simulink model "MultiAgentNewtonian"  (R2017a)
settings: Solver=ode1  StartTime=0.0  StopTime=50  FixedStep=tstep  RelTol=1e-3
InitFcn:
  | initSim;
StopFcn:
  | plotSimSolution;
values from neighbouring files (symbols this model uses):
  tstep = 0.1    [initSim.m]
undefined symbols (not defined in the file or in its folder): m, problem
settings Model: Creator=yn15  LastModifiedBy=DAW15
settings OptimizationCC: LifeSpan=inf
settings DebuggingCC: SFUnexpectedBacktrackingDiag=warning  SFNoUnconditionalDefaultTransitionDiag=warning  SFExecutionAtInitializationDiag=none
settings GRTTargetCC: TargetLangStandard=C89/C90 (ANSI)
settings ConfigComp: CovMetricSettings=dw  CovHtmlReporting=on  CovSaveCumulativeToWorkspaceVar=on  CovSaveSingleToWorkspaceVar=on  CovExternalEMLEnable=off

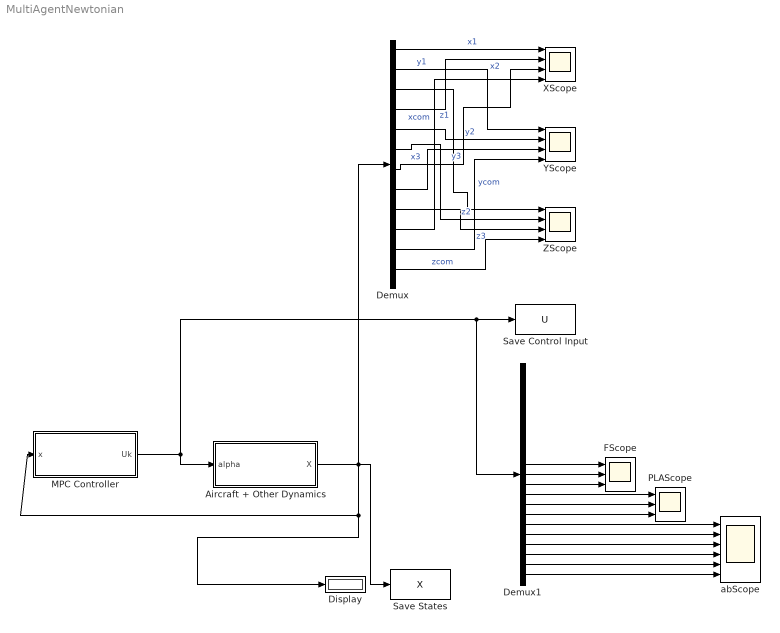
== system MultiAgentNewtonian ==
  Aircraft + Other Dynamics : Subsystem
  Demux : Demux  Outputs=24
  Demux1 : Demux  Outputs=21
  Display : Display
  FScope : Scope  NumInputPorts=3
  "MPC Controller " : Subsystem
  PLAScope : Scope  NumInputPorts=3
  Save Control Input : ToWorkspace  VariableName=U  SampleTime=-1
      settings: Save2DSignal=2-D array (concatenate along first dimension)
  Save States : ToWorkspace  VariableName=X  SaveFormat=Timeseries  SampleTime=-1
  XScope : Scope  NumInputPorts=4
  YScope : Scope  NumInputPorts=4
  ZScope : Scope  NumInputPorts=4
  abScope : Scope  NumInputPorts=6
  wires:
  Aircraft + Other Dynamics/1(X) -> Demux/1, Save States/1, "MPC Controller "/1(x), Display/1
  "MPC Controller "/1(Uk) -> Demux1/1, Save Control Input/1, Aircraft + Other Dynamics/1(alpha)
  Demux/1 -> XScope/1  "x1"
  Demux/3 -> YScope/1  "y1"
  Demux/5 -> ZScope/1  "z1"
  Demux/7 -> XScope/2  "x2"
  Demux/9 -> YScope/2  "y2"
  Demux/11 -> ZScope/2  "z2"
  Demux/13 -> XScope/3  "x3"
  Demux/15 -> YScope/3  "y3"
  Demux/17 -> ZScope/3  "z3"
  Demux/19 -> XScope/4  "xcom"
  Demux/21 -> YScope/4  "ycom"
  Demux/23 -> ZScope/4  "zcom"
  Demux1/10 -> FScope/1
  Demux1/11 -> FScope/2
  Demux1/12 -> FScope/3
  Demux1/13 -> PLAScope/1
  Demux1/14 -> PLAScope/2
  Demux1/15 -> PLAScope/3
  Demux1/16 -> abScope/1
  Demux1/17 -> abScope/2
  Demux1/18 -> abScope/3
  Demux1/19 -> abScope/4
  Demux1/20 -> abScope/5
  Demux1/21 -> abScope/6

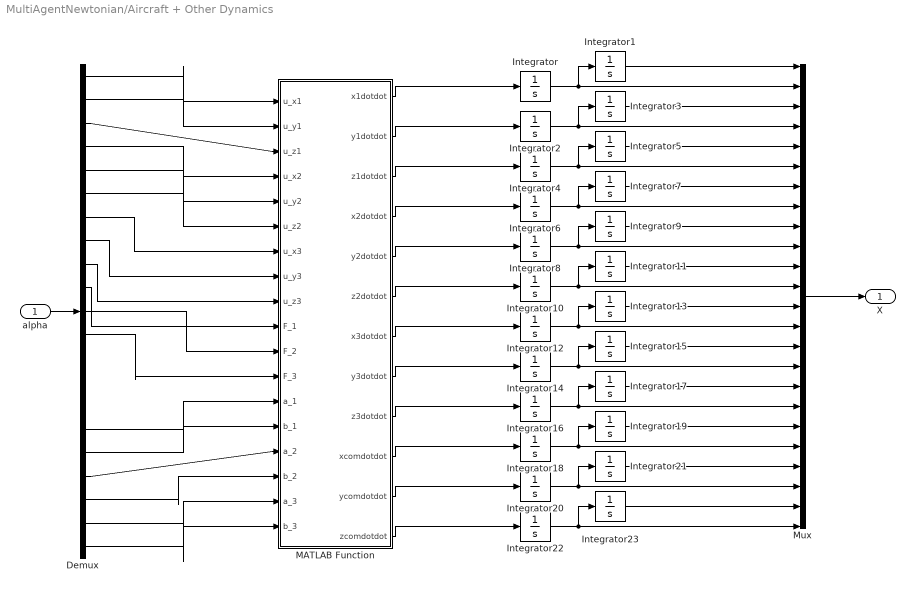
== system MultiAgentNewtonian/Aircraft + Other Dynamics ==
  alpha : Inport
  Demux : Demux  Outputs=21
  Integrator{,1..23} (24 alike) : Integrator
  MATLAB Function : MATLAB Function  TreatAsAtomicUnit=on
  Mux : Mux  Inputs=24
  X : Outport
  wires:
  MATLAB Function/3(z1dotdot) -> Integrator4/1
  MATLAB Function/6(z2dotdot) -> Integrator10/1
  MATLAB Function/9(z3dotdot) -> Integrator16/1
  Integrator/1 -> Mux/2, Integrator1/1
  MATLAB Function/1(x1dotdot) -> Integrator/1
  Integrator2/1 -> Mux/4, Integrator3/1
  Integrator4/1 -> Mux/6, Integrator5/1
  Integrator6/1 -> Mux/8, Integrator7/1
  Integrator8/1 -> Mux/10, Integrator9/1
  Integrator10/1 -> Mux/12, Integrator11/1
  Integrator12/1 -> Mux/14, Integrator13/1
  Integrator14/1 -> Mux/16, Integrator15/1
  Integrator16/1 -> Mux/18, Integrator17/1
  Integrator18/1 -> Mux/20, Integrator19/1
  Integrator20/1 -> Mux/22, Integrator21/1
  Integrator22/1 -> Mux/24, Integrator23/1
  MATLAB Function/2(y1dotdot) -> Integrator2/1
  MATLAB Function/4(x2dotdot) -> Integrator6/1
  MATLAB Function/5(y2dotdot) -> Integrator8/1
  MATLAB Function/7(x3dotdot) -> Integrator12/1
  MATLAB Function/8(y3dotdot) -> Integrator14/1
  MATLAB Function/10(xcomdotdot) -> Integrator18/1
  MATLAB Function/11(ycomdotdot) -> Integrator20/1
  MATLAB Function/12(zcomdotdot) -> Integrator22/1
  Integrator1/1 -> Mux/1
  Integrator3/1 -> Mux/3
  Integrator5/1 -> Mux/5
  Integrator7/1 -> Mux/7
  Integrator9/1 -> Mux/9
  Integrator11/1 -> Mux/11
  Integrator13/1 -> Mux/13
  Integrator15/1 -> Mux/15
  Integrator17/1 -> Mux/17
  Integrator19/1 -> Mux/19
  Integrator21/1 -> Mux/21
  Integrator23/1 -> Mux/23
  Mux/1 -> X/1
  alpha/1 -> Demux/1
  Demux/1 -> MATLAB Function/1(u_x1)
  Demux/2 -> MATLAB Function/2(u_y1)
  Demux/3 -> MATLAB Function/3(u_z1)
  Demux/4 -> MATLAB Function/4(u_x2)
  Demux/5 -> MATLAB Function/5(u_y2)
  Demux/6 -> MATLAB Function/6(u_z2)
  Demux/7 -> MATLAB Function/7(u_x3)
  Demux/8 -> MATLAB Function/8(u_y3)
  Demux/9 -> MATLAB Function/9(u_z3)
  Demux/10 -> MATLAB Function/10(F_1)
  Demux/11 -> MATLAB Function/11(F_2)
  Demux/12 -> MATLAB Function/12(F_3)
  Demux/16 -> MATLAB Function/13(a_1)
  Demux/17 -> MATLAB Function/14(b_1)
  Demux/18 -> MATLAB Function/15(a_2)
  Demux/19 -> MATLAB Function/16(b_2)
  Demux/20 -> MATLAB Function/17(a_3)
  Demux/21 -> MATLAB Function/18(b_3)

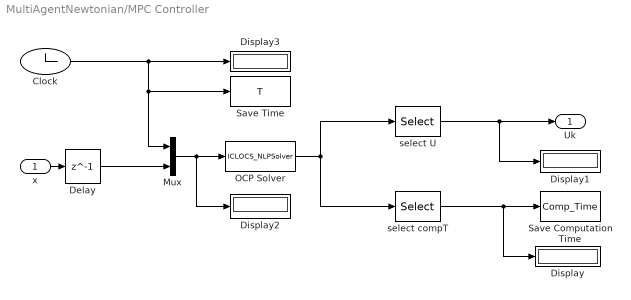
== system MultiAgentNewtonian/MPC Controller  ==
  x : Inport
  Clock : Clock
  Delay : Delay  DelayLength=1  InitialCondition=[problem.states.x0]
  Display{,1..3} (4 alike) : Display
  Mux : Mux  Inputs=2
  OCP Solver : MATLABFcn  MATLABFcn=ICLOCS_NLPSolver  OutputDimensions=m+2
  "Save Computation Time " : ToWorkspace  VariableName=Comp_Time  SampleTime=tstep
      settings: Save2DSignal=2-D array (concatenate along first dimension)
  Save Time : ToWorkspace  VariableName=T  SampleTime=-1
      settings: Save2DSignal=2-D array (concatenate along first dimension)
  select U : Selector  IndexOptions=Index vector (dialog)  Indices=3:m+2  OutputSizes=1
  select compT : Selector  IndexOptions=Index vector (dialog)  Indices=2  OutputSizes=1
  Uk : Outport
  wires:
  select U/1 -> Display1/1, Uk/1
  x/1 -> Delay/1
  OCP Solver/1 -> select U/1, select compT/1
  Clock/1 -> Save Time/1, Mux/1, Display3/1
  select compT/1 -> Display/1, "Save Computation Time "/1
  Mux/1 -> Display2/1, OCP Solver/1
  Delay/1 -> Mux/2

== matlab function MultiAgentNewtonian/Aircraft + Other Dynamics/MATLAB Function ==
  data: x1dotdot output; u_x1 input; u_y1 input; u_z1 input; u_x2 input; u_y2 input; u_z2 input; u_x3 input; u_y3 input; u_z3 input; y1dotdot output; z1dotdot output; x2dotdot output; y2dotdot output; z2dotdot output; x3dotdot output; y3dotdot output; z3dotdot output; xcomdotdot output; ycomdotdot output; zcomdotdot output; F_1 input; F_2 input; F_3 input; a_1 input; b_1 input; a_2 input; b_2 input; a_3 input; b_3 input
function [x1dotdot,y1dotdot,z1dotdot,...
    x2dotdot,y2dotdot,z2dotdot,x3dotdot,y3dotdot,z3dotdot,...
    xcomdotdot,ycomdotdot,zcomdotdot]= fcn(u_x1,u_y1,u_z1,u_x2,u_y2,u_z2,u_x3,u_y3,u_z3,F_1,F_2,F_3,a_1,b_1,a_2,b_2,a_3,b_3)

m_ag = 0.81;
m_pl = 20;
g = 9.81;

x1dotdot = (1/m_ag)*(u_x1-F_1*tan(a_1)); %x1..
y1dotdot = (1/m_ag)*(u_y1 - F_1*tan(b_1)); %y1..
z1dotdot = (1/m_ag)*(u_z1 - F_1 - m_ag*g); %z1..
x2dotdot = (1/m_ag)*(u_x2 - F_2*tan(a_2)); %x2..
y2dotdot = (1/m_ag)*(u_y2 - F_2*tan(b_2)); %y2..
z2dotdot = (1/m_ag)*(u_z2 - F_2 - m_ag*g); %z2..
x3dotdot = (1/m_ag)*(u_x3 - F_3*tan(a_3)); %x3..
y3dotdot = (1/m_ag)*(u_y3 - F_3*tan(b_3)); %y3..
z3dotdot = (1/m_ag)*(u_z3 - F_3 - m_ag*g); %z3..
xcomdotdot =  (1/m_pl)*(u_x1+u_x2+u_x3 - m_ag*(x1dotdot+x2dotdot+x3dotdot));%xcom..
ycomdotdot =  (1/m_pl)*(u_y1+u_y2+u_y3 - m_ag*(y1dotdot+y2dotdot+y3dotdot));%ycom..
zcomdotdot =  (1/m_pl)*(u_z1+u_z2+u_z3 - m_ag*(z1dotdot+z2dotdot+z3dotdot - 3*g));%zcom..
